simulink model "Temp2"  (Simulink 7.7)
settings: Solver=ode45  StartTime=0.0  StopTime=10.0  RelTol=1e-3
undefined symbols (not defined in the file or in its folder): gray
libraries: vipsnks x3, dspmtrx3 x2, simulink x1, dspsnks4 x1, vipconversions x1, vipsrcs x1
settings Model: Creator=katsikas  LastModifiedBy=katsikas

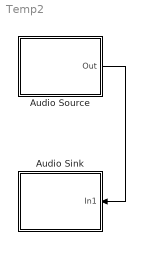
== system Temp2 ==
  Audio Sink : Subsystem
  Audio Source : Subsystem
  wires:
  Audio Source/1(Out) -> Audio Sink/1(In1)

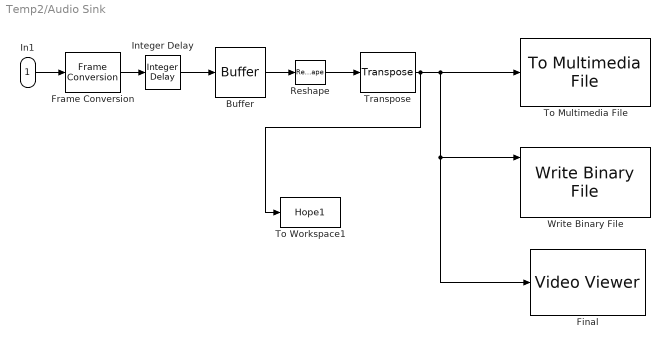
== system Temp2/Audio Sink ==
  In1 : Inport
  Buffer : Buffer  N=19200  TreatMby1Signals=One channel
  Final : vipsnks/Video Viewer  inputType=Obsolete7b  imagePorts=One multidimensional signal  useColorMap=off  colormapValue=gray(256)  specRange=off  minInputVal=0  maxInputVal=255  FigPos=[749 1039 506 522]  AxisZoom=on  trueSizedOnce=on  OpenAtMdlStart=on
  Frame Conversion : FrameConversion  OutFrame=Sample-based
  Integer Delay : simulink/Discrete/Integer Delay  NumDelays=180  vinit=0.0  samptime=-1
  Reshape : Reshape  OutputDimensionality=Customize  OutputDimensions=[160,120]
  To Multimedia File : dspsnks4/To Multimedia File  outputFilename=output.avi  streamSelection=Video only  videoCompressor=None (uncompressed)  audioCompressor=None (uncompressed)  imagePorts=One multidimensional signal  fileType=AVI  audioDatatype=Determine from input data type  fourcc=RGB
  To Workspace1 : ToWorkspace  VariableName=Hope1  SampleTime=-1  SaveFormat=Array
      settings: MaxDataPoints=10000
  Transpose : dspmtrx3/Transpose  SystemSampleTime=-1  Hermitian=off  overflowFlag=off
  Write Binary File : vipsnks/Write Binary File  FileName=output.bin  VideoFormat=Four character codes  FOURCC=I420  BitStreamFormat=Planar  NumInputs=3  ComponentOrder=[1 2 3]  Interlaced=off  LineOrdering=Top line first  InheritBits=on  Component1=Y'  Component2=Cb  Component3=Cr  Component4=Alpha  Bits1=8  Bits2=8  Bits3=8  Bits4=0  SignedInput=off  FileEndian=Little endian
  wires:
  Reshape/1 -> Transpose/1
  In1/1 -> Frame Conversion/1
  Transpose/1 -> To Multimedia File/1, Final/1, Write Binary File/1, To Workspace1/1
  Buffer/1 -> Reshape/1
  Integer Delay/1 -> Buffer/1
  Frame Conversion/1 -> Integer Delay/1

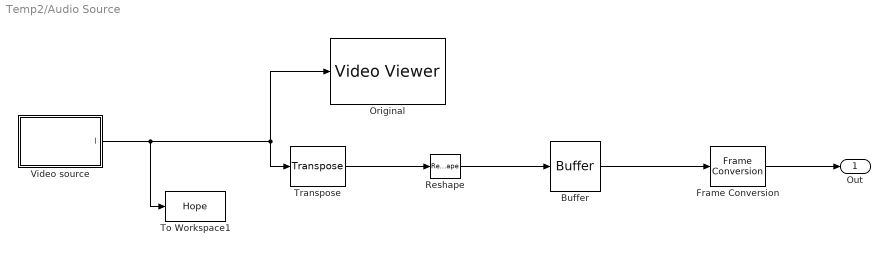
== system Temp2/Audio Source ==
  Buffer : Buffer  N=188  TreatMby1Signals=One channel
  Frame Conversion : FrameConversion
  Original : vipsnks/Video Viewer  inputType=Obsolete7b  imagePorts=One multidimensional signal  useColorMap=off  colormapValue=gray(256)  specRange=off  minInputVal=0  maxInputVal=255  FigPos=[32 1021 682 887]  AxisZoom=on  trueSizedOnce=on  OpenAtMdlStart=on
  Reshape : Reshape
  To Workspace1 : ToWorkspace  VariableName=Hope  SampleTime=-1  SaveFormat=Array
      settings: MaxDataPoints=10000
  Transpose : dspmtrx3/Transpose  SystemSampleTime=-1  Hermitian=off  overflowFlag=off
  Video source : Subsystem
  Out : Outport
  wires:
  Reshape/1 -> Buffer/1
  Video source/1(I) -> Original/1, Transpose/1, To Workspace1/1
  Transpose/1 -> Reshape/1
  Buffer/1 -> Frame Conversion/1
  Frame Conversion/1 -> Out/1

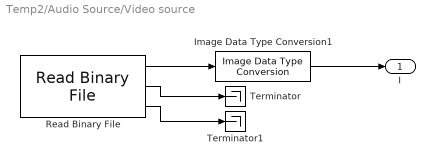
== system Temp2/Audio Source/Video source ==
  Image Data Type Conversion1 : vipconversions/Image Data Type Conversion  outDT=uint8  isSigned=on  wordLen=16  numFracBits=0
  Read Binary File : vipsrcs/Read Binary File  FileName=vipmen.bin  loopOrNot=on  numLoops=inf  VideoFormat=Custom  FOURCC=I420  BitStreamFormat=Planar  NumOutputs=3  ComponentOrder=[1 2 3]  Interlaced=off  LineOrdering=Top line first  Ts=1/30  Component1=Y'  Component2=Cb  Component3=Cr  Component4=Alpha  Bits1=8  Bits2=8  Bits3=8  Bits4=8  Rows1=120  Rows2=60  Rows3=60  Rows4=288  Cols1=160  Cols2=80  Cols3=80  Cols4=352  YRows=288  YCols=352  SignedOutput=off  FileEndian=Little endian  OutputEOF=off
  Terminator : Terminator
  Terminator1 : Terminator
  I : Outport
  wires:
  Image Data Type Conversion1/1 -> I/1
  Read Binary File/1 -> Image Data Type Conversion1/1
  Read Binary File/2 -> Terminator/1
  Read Binary File/3 -> Terminator1/1
